simulink model "Hysteresis_transition"  (R2020b)
settings: Solver=VariableStepAuto  StartTime=0.0  StopTime=10.0  RelTol=1e-3
settings Model: Creator=Training  LastModifiedBy=Training

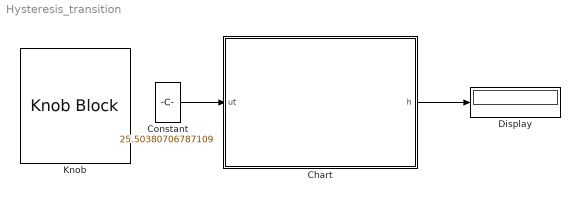
== system Hysteresis_transition ==
  Chart : Stateflow chart  TreatAsAtomicUnit=on
  Constant : Constant  Value=25.50380706787109
  Display : Display
  Knob : KnobBlock
  wires:
  Constant/1 -> Chart/1(ut)
  Chart/1(h) -> Display/1

== stateflow chart Hysteresis_transition/Chart ==
  (default) -> (junction 5) : {at=18;,delta=2;}
  (junction 5) -> (junction 2) [order 1] : [at>ut &&at-ut >= delta]
  (junction 5) -> (junction 14) [order 2]
  (junction 2) -> (junction 7) : {h=-1;}
  (junction 14) -> (junction 4) [order 1] : [at<ut && ut-at >=delta]
  (junction 14) -> (junction 3) [order 2] : {h=0;}
  (junction 4) -> (junction 6) : {h=1;}
  (junction 6) -> (junction 3)
  (junction 7) -> (junction 6)
  (junction 3) -> (junction 8)
  data: at local; ut input; delta local; h output
